simulink model "control_posicion_cascada"  (Simulink 8.5)
settings: Solver=ode45  StartTime=0.0  StopTime=30  RelTol=1e-3
values from neighbouring files (symbols this model uses):
  Hz = 10    [modelo_controlador_analisis.m]
  T = 0.02    [modelo_controlador_analisis.m]
libraries: simulink x2
settings Model: Creator=ARTURO  LastModifiedBy=ARTURO
settings DataIOCC: SignalLoggingSaveFormat=Dataset
settings OptimizationCC: ExpressionDepthLimit=128
settings DebuggingCC: UnderspecifiedInitializationDetection=Simplified  MergeDetectMultiDrivingBlocksExec=error  FcnCallInpInsideContextMsg=EnableAllAsError  StateNameClashWarn=none
settings GRTTargetCC: CombineOutputUpdateFcns=on  GRTInterface=off

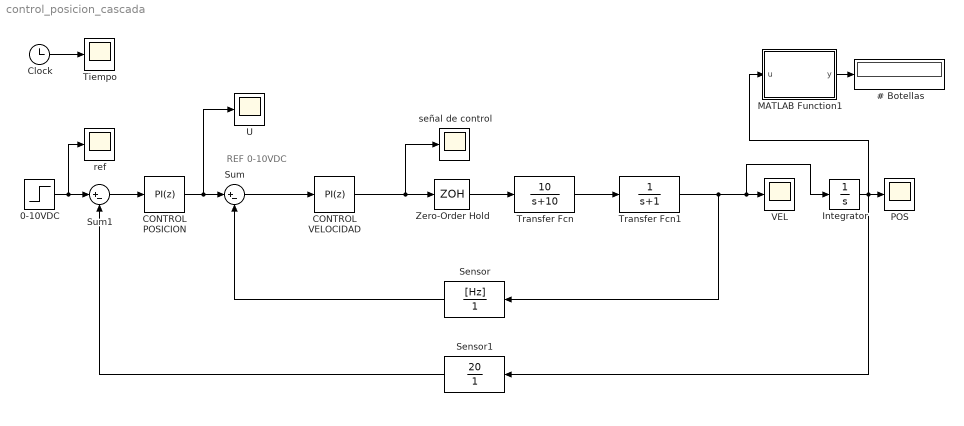
== system control_posicion_cascada ==
  note: REF 0-10VDC
  # Botellas : Display
  0-10VDC : Step  Time=0  After=10  SampleTime=0
  CONTROL POSICION : simulink/Continuous/PID Controller  Controller=PI  TimeDomain=Discrete-time  SampleTime=T  IntegratorMethod=Trapezoidal  FilterMethod=Forward Euler  Form=Parallel  UseFilter=on  ControllerParametersSource=internal  P=1.08996277463501  I=0.0412763969334678  D=0.444515782433963  N=90.4582395590637  InitialConditionSource=internal  InitialConditionForIntegrator=0  InitialConditionForFilter=0  ExternalReset=none  LimitOutput=off  UpperSaturationLimit=inf  LowerSaturationLimit=-inf  LinearizeAsGain=off  AntiWindupMode=none  Kb=1  TrackingMode=off  Kt=1  PParamMin=[]  PParamMax=[]  IParamMin=[]  IParamMax=[]  DParamMin=[]  DParamMax=[]  NParamMin=[]  NParamMax=[]  KbParamMin=[]  KbParamMax=[]  KtParamMin=[]  KtParamMax=[]  POutMin=[]  POutMax=[]  IOutMin=[]  IOutMax=[]  DOutMin=[]  DOutMax=[]  NOutMin=[]  NOutMax=[]  KbOutMin=[]  KbOutMax=[]  KtOutMin=[]  KtOutMax=[]  IntegratorOutMin=[]  IntegratorOutMax=[]  FilterOutMin=[]  FilterOutMax=[]  SumOutMin=[]  SumOutMax=[]  SumI1OutMin=[]  SumI1OutMax=[]  SumI2OutMin=[]  SumI2OutMax=[]  SumI3OutMin=[]  SumI3OutMax=[]  SumDOutMin=[]  SumDOutMax=[]  SaturationOutMin=[]  SaturationOutMax=[]  IntegratorContinuousStateAttributes=''  IntegratorStateMustResolveToSignalObject=off  IntegratorRTWStateStorageClass=Auto  FilterContinuousStateAttributes=''  FilterStateMustResolveToSignalObject=off  FilterRTWStateStorageClass=Auto  DifferentiatorICPrevScaledInput=0  DifferentiatorOutMin=[]  DifferentiatorOutMax=[]
  "CONTROL VELOCIDAD " : simulink/Continuous/PID Controller  Controller=PI  TimeDomain=Discrete-time  SampleTime=T  IntegratorMethod=Trapezoidal  FilterMethod=Forward Euler  Form=Parallel  UseFilter=on  ControllerParametersSource=internal  P=0.8511  I=0.5881  D=0  N=100  InitialConditionSource=internal  InitialConditionForIntegrator=0  InitialConditionForFilter=0  ExternalReset=none  LimitOutput=off  UpperSaturationLimit=inf  LowerSaturationLimit=-inf  LinearizeAsGain=off  AntiWindupMode=none  Kb=1  TrackingMode=off  Kt=1  PParamMin=[]  PParamMax=[]  IParamMin=[]  IParamMax=[]  DParamMin=[]  DParamMax=[]  NParamMin=[]  NParamMax=[]  KbParamMin=[]  KbParamMax=[]  KtParamMin=[]  KtParamMax=[]  POutMin=[]  POutMax=[]  IOutMin=[]  IOutMax=[]  DOutMin=[]  DOutMax=[]  NOutMin=[]  NOutMax=[]  KbOutMin=[]  KbOutMax=[]  KtOutMin=[]  KtOutMax=[]  IntegratorOutMin=[]  IntegratorOutMax=[]  FilterOutMin=[]  FilterOutMax=[]  SumOutMin=[]  SumOutMax=[]  SumI1OutMin=[]  SumI1OutMax=[]  SumI2OutMin=[]  SumI2OutMax=[]  SumI3OutMin=[]  SumI3OutMax=[]  SumDOutMin=[]  SumDOutMax=[]  SaturationOutMin=[]  SaturationOutMax=[]  IntegratorContinuousStateAttributes=''  IntegratorStateMustResolveToSignalObject=off  IntegratorRTWStateStorageClass=Auto  FilterContinuousStateAttributes=''  FilterStateMustResolveToSignalObject=off  FilterRTWStateStorageClass=Auto  DifferentiatorICPrevScaledInput=0  DifferentiatorOutMin=[]  DifferentiatorOutMax=[]
  Clock : Clock
  Integrator : Integrator
  MATLAB Function1 : MATLAB Function  TreatAsAtomicUnit=on
  "POS " : Scope
      settings: TimeRange=100  YMin=0  YMax=0.6000000000000001  SaveName=pos
  Sensor : DiscreteTransferFcn  Numerator=[Hz]  Denominator=[1]  SampleTime=T
  Sensor1 : DiscreteTransferFcn  Numerator=[20]  Denominator=[1]  SampleTime=T
  Sum : Sum  Inputs=|+-
  Sum1 : Sum  Inputs=|+-
  "Tiempo " : Scope
      settings: YMin=-1.25  YMax=11.25  SaveName=tiempo
  Transfer Fcn : TransferFcn  Numerator=[10]  Denominator=[1 10]
  Transfer Fcn1 : TransferFcn  Denominator=[1 1]
  U : Scope
  "VEL " : Scope
      settings: YMin=-0.01406  YMax=0.12652  SaveName=y
  Zero-Order Hold : ZeroOrderHold  SampleTime=T
  ref : Scope
      settings: TimeRange=20  YMin=0  YMax=2.5  SaveName=r
  señal de control : Scope
      settings: YMin=-0.13264  YMax=0.96694  SaveName=u
  wires:
  Transfer Fcn1/1 -> Sensor/1, Integrator/1, "VEL "/1
  Sum/1 -> "CONTROL VELOCIDAD "/1
  Zero-Order Hold/1 -> Transfer Fcn/1
  Transfer Fcn/1 -> Transfer Fcn1/1
  Sensor/1 -> Sum/2
  "CONTROL VELOCIDAD "/1 -> señal de control/1, Zero-Order Hold/1
  Clock/1 -> "Tiempo "/1
  0-10VDC/1 -> Sum1/1, ref/1
  MATLAB Function1/1(y) -> # Botellas/1
  CONTROL POSICION/1 -> U/1, Sum/1
  Integrator/1 -> Sensor1/1, MATLAB Function1/1(u), "POS "/1
  Sum1/1 -> CONTROL POSICION/1
  Sensor1/1 -> Sum1/2

== matlab function MATLAB Function1 ==
  data: u input double; y output double
function y = fcn(u)

y = u/0.5;

y = 5*ceil(y);
